simulink model "FF_Controller"  (R2022b)
settings: Solver=VariableStepAuto  StartTime=0.0  StopTime=10.0  RelTol=1e-3
libraries: ros2lib x8, matrix_library x1

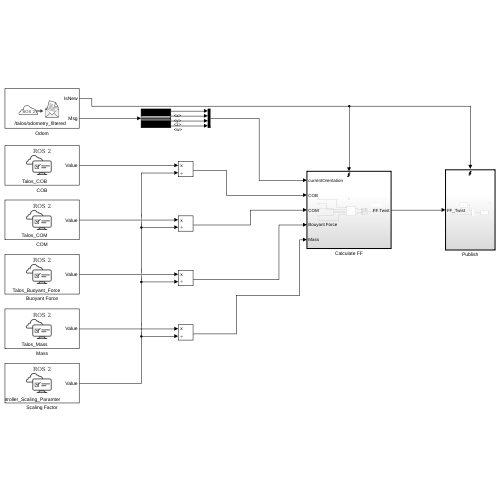
[thumbnail: Simulink's stored preview of the top-level diagram]
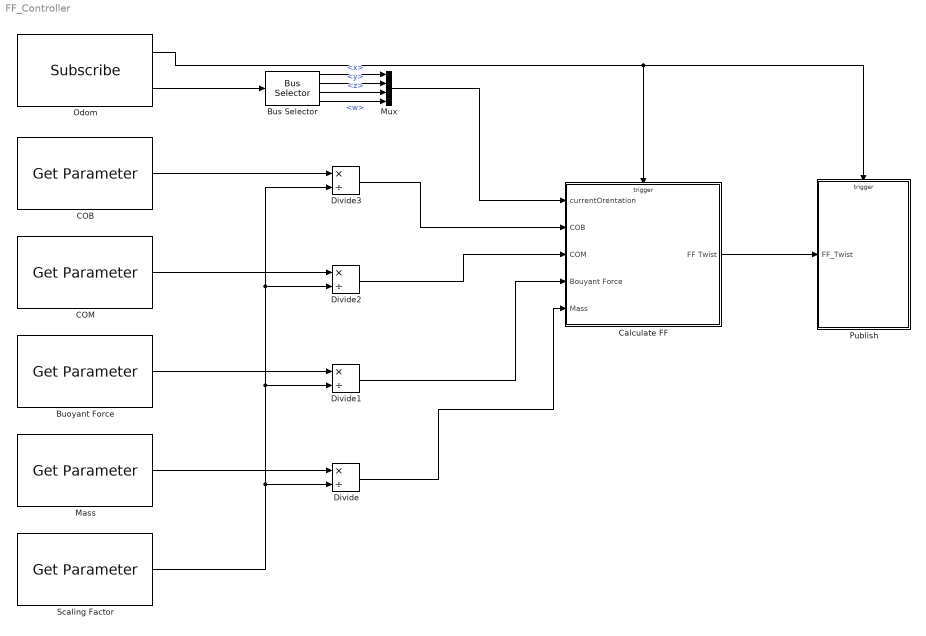
== system FF_Controller ==
  Buoyant Force : ros2lib/Get Parameter  ParameterName=Talos_Buoyant_Force  ParameterType=double  ParameterMaxArrayLength=16  ParameterInitialValue=0.0  SampleTime=-1  ModelName=FF_Controller  BlockId=ParamGet_FF_Controller_69
  Bus Selector : BusSelector  OutputSignals=pose.pose.orientation.x,pose.pose.orientation.y,pose.pose.orientation.z,pose.pose.orientation.w
  COB : ros2lib/Get Parameter  ParameterName=Talos_COB  ParameterType=double  ParameterMaxArrayLength=16  ParameterInitialValue=0.0  SampleTime=-1  ModelName=FF_Controller  BlockId=ParamGet_FF_Controller_67
  COM : ros2lib/Get Parameter  ParameterName=Talos_COM  ParameterType=double  ParameterMaxArrayLength=16  ParameterInitialValue=0.0  SampleTime=-1  ModelName=FF_Controller  BlockId=ParamGet_FF_Controller_68
  Calculate FF : Subsystem
  Divide{,1..3} (4 alike) : Product  Inputs=*/
  Mass : ros2lib/Get Parameter  ParameterName=Talos_Mass  ParameterType=double  ParameterMaxArrayLength=16  ParameterInitialValue=0.0  SampleTime=-1  ModelName=FF_Controller  BlockId=ParamGet_FF_Controller_70
  Mux : Mux
  Odom : ros2lib/Subscribe  topicSource=Specify your own  topic=/talos/odometry_filtered  messageType=nav_msgs/Odometry  sampleTime=-1  QOSHistory=Keep last  QOSDepth=1  QOSReliability=Reliable  QOSDurability=Volatile
  Publish : Subsystem
  Scaling Factor : ros2lib/Get Parameter  ParameterName=FF_Controller_Scaling_Paramter  ParameterType=int64  ParameterMaxArrayLength=16  ParameterInitialValue=1  SampleTime=-1  ModelName=FF_Controller  BlockId=ParamGet_FF_Controller_71
  wires:
  Calculate FF/1(FF Twist) -> Publish/1(FF_Twist)
  Odom/2 -> Bus Selector/1
  Odom/1 -> Publish/Trigger, Calculate FF/Trigger
  Bus Selector/1 -> Mux/1  "<x>"
  Bus Selector/2 -> Mux/2  "<y>"
  Bus Selector/3 -> Mux/3  "<z>"
  Bus Selector/4 -> Mux/4  "<w>"
  Mux/1 -> Calculate FF/1(currentOrentation)
  COM/1 -> Divide2/1
  Buoyant Force/1 -> Divide1/1
  Mass/1 -> Divide/1
  COB/1 -> Divide3/1
  Divide3/1 -> Calculate FF/2(COB)
  Divide2/1 -> Calculate FF/3(COM)
  Divide1/1 -> Calculate FF/4(Bouyant Force)
  Divide/1 -> Calculate FF/5(Mass)
  Scaling Factor/1 -> Divide3/2, Divide2/2, Divide1/2, Divide/2

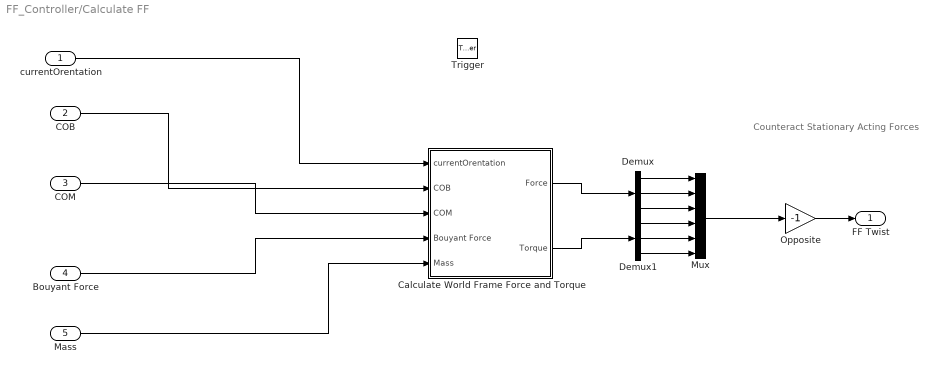
== system FF_Controller/Calculate FF ==
  note: Counteract Stationary Acting Forces
  currentOrentation : Inport
  COB : Inport  Port=2
  COM : Inport  Port=3
  Bouyant Force : Inport  Port=4
  Mass : Inport  Port=5
  Trigger : TriggerPort  VariantControl=(inherit)  PortDimensions=1
  Calculate World Frame Force and Torque : Subsystem
  Demux : Demux  Outputs=3
  Demux1 : Demux  Outputs=3
  Mux : Mux  Inputs=6
  Opposite : Gain  Gain=-1
  FF Twist : Outport
  wires:
  Calculate World Frame Force and Torque/1(Force) -> Demux/1
  Opposite/1 -> FF Twist/1
  currentOrentation/1 -> Calculate World Frame Force and Torque/1(currentOrentation)
  Demux1/2 -> Mux/5
  COM/1 -> Calculate World Frame Force and Torque/3(COM)
  Demux/2 -> Mux/2
  Mux/1 -> Opposite/1
  Calculate World Frame Force and Torque/2(Torque) -> Demux1/1
  COB/1 -> Calculate World Frame Force and Torque/2(COB)
  Demux/1 -> Mux/1
  Demux1/3 -> Mux/6
  Demux1/1 -> Mux/4
  Demux/3 -> Mux/3
  Mass/1 -> Calculate World Frame Force and Torque/5(Mass)
  Bouyant Force/1 -> Calculate World Frame Force and Torque/4(Bouyant Force)

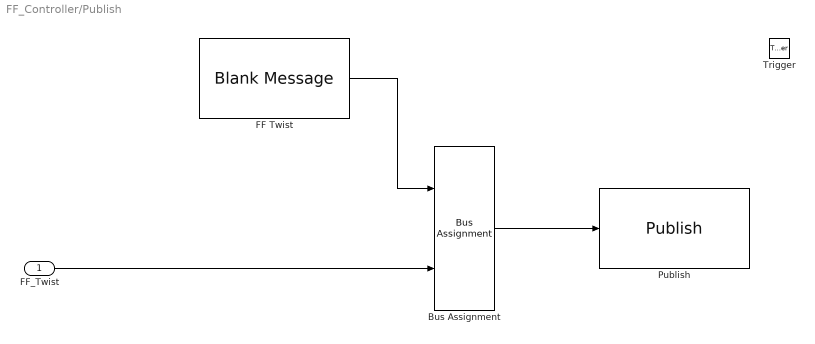
== system FF_Controller/Publish ==
  FF_Twist : Inport
  Trigger : TriggerPort  VariantControl=(inherit)  PortDimensions=1
  Bus Assignment : BusAssignment  AssignedSignals=signal1
  FF Twist : ros2lib/Blank Message  messageClass=Message  entityType=geometry_msgs/Twist  messageType=geometry_msgs/Twist  SampleTime=inf
  Publish : ros2lib/Publish  topicSource=Specify your own  topic=/talos/controller/FF_body_force  messageType=geometry_msgs/Point  QOSHistory=Keep last  QOSDepth=1  QOSReliability=Reliable  QOSDurability=Volatile
  wires:
  Bus Assignment/1 -> Publish/1
  FF Twist/1 -> Bus Assignment/1
  FF_Twist/1 -> Bus Assignment/2

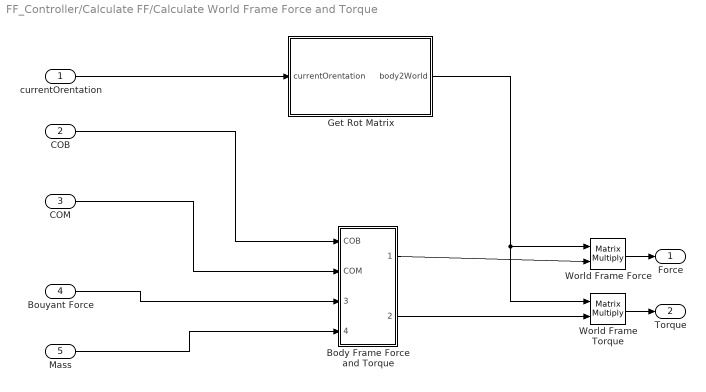
== system FF_Controller/Calculate FF/Calculate World Frame Force and Torque ==
  currentOrentation : Inport
  COB : Inport  Port=2
  COM : Inport  Port=3
  Bouyant Force : Inport  Port=4
  Mass : Inport  Port=5
  Body Frame Force and Torque : Subsystem
  Get Rot Matrix : MATLAB Function  TreatAsAtomicUnit=on
  World Frame Force : Product  Multiplication=Matrix(*)
  World Frame Torque : Product  Multiplication=Matrix(*)
  Force : Outport
  Torque : Outport  Port=2
  wires:
  Body Frame Force and Torque/1(force) -> World Frame Force/2
  World Frame Force/1 -> Force/1
  Get Rot Matrix/1(body2World) -> World Frame Torque/1, World Frame Force/1
  Bouyant Force/1 -> Body Frame Force and Torque/3(Bouyant Force)
  COM/1 -> Body Frame Force and Torque/2(COM)
  COB/1 -> Body Frame Force and Torque/1(COB)
  Body Frame Force and Torque/2(torque) -> World Frame Torque/2
  currentOrentation/1 -> Get Rot Matrix/1(currentOrentation)
  Mass/1 -> Body Frame Force and Torque/4(Mass)
  World Frame Torque/1 -> Torque/1

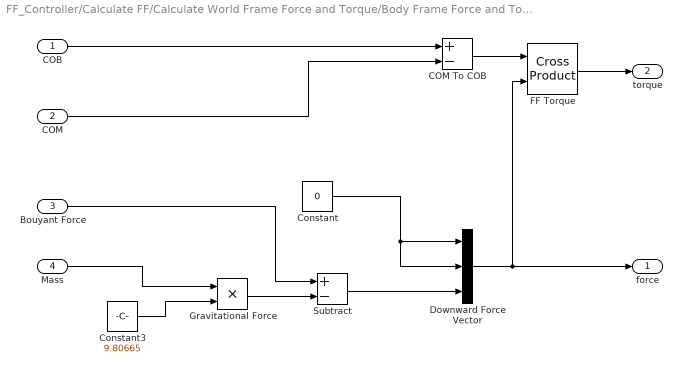
== system FF_Controller/Calculate FF/Calculate World Frame Force and Torque/Body Frame Force and Torque ==
  COB : Inport
  COM : Inport  Port=2
  Bouyant Force : Inport  Port=3
  Mass : Inport  Port=4
  COM To COB : Sum  Inputs=+-
  Constant : Constant  Value=0
  Constant3 : Constant  Value=9.80665
  Downward Force Vector : Mux  Inputs=3
  FF Torque : matrix_library/Cross Product
  Gravitational Force : Product
  Subtract : Sum  Inputs=+-
  force : Outport
  torque : Outport  Port=2
  wires:
  COM To COB/1 -> FF Torque/1
  Constant/1 -> Downward Force Vector/1, Downward Force Vector/2
  Downward Force Vector/1 -> force/1, FF Torque/2
  Subtract/1 -> Downward Force Vector/3
  Gravitational Force/1 -> Subtract/2
  COM/1 -> COM To COB/2
  FF Torque/1 -> torque/1
  COB/1 -> COM To COB/1
  Constant3/1 -> Gravitational Force/2
  Mass/1 -> Gravitational Force/1
  Bouyant Force/1 -> Subtract/1

== matlab function FF_Controller/Calculate FF/Calculate World Frame Force and Torque/Get Rot Matrix ==
function body2World = fcn(currentOrentation)

%change ros quat to matlab quat
quat = [currentOrentation(4), currentOrentation(1), currentOrentation(2), currentOrentation(3)];

%generate world to body rotation matrix
world2body = quat2rotm(quat);

%inv rot = transpose rot
body2World = transpose(world2body);
